simulink model "CT_tests_2020b"  (R2020b)
settings: Solver=ode4  StartTime=0.0  StopTime=0.4  FixedStep=10e-6  RelTol=1e-3
libraries: CT_RTDS x1, spsControlledCurrentSourceLib x1, spsSeriesRLCBranchLib x1, spspowerguiLib x1
settings Model: SimulationMode=accelerator  Creator=valeriytashchilin  LastModifiedBy=valeriytashchilin
settings DataIOCC: SaveOutput=off  SignalLogging=off  DSMLogging=off  SaveTime=off  ReturnWorkspaceOutputs=off

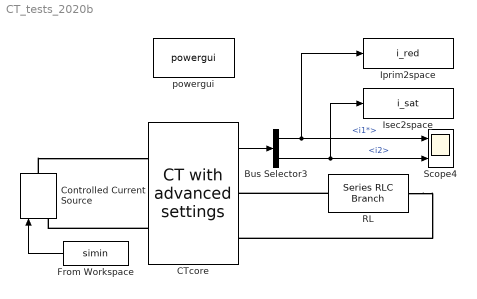
== system CT_tests_2020b ==
  Bus Selector3 : BusSelector  OutputSignals=i1*,i2
  CTcore : CT_RTDS/CT with advanced settings  Tag=CT  N1=2  N2=239  R2=0.48  L2=0  D=100  S=19.1e-4  Length=90e-2  Rloss=1e12  B0=0  c=0.08  k=4e-5  BETA1=0.96  ALFA=3e-5  Ms=1.7e6  a1=2550  a2=3150  a3=15000  b=2  SIMPLE=on  H2=600  DSCR=on  ts=-1  BAL=off
      settings: SourceProductName=CT RTDS
  Controlled Current Source : spsControlledCurrentSourceLib/Controlled Current Source  Initialize=on  Source_Type=AC  Amplitude=0  Phase=0  Frequency=0  Measurements=None
  From Workspace : FromWorkspace  VariableName=simin
  Iprim2space : ToWorkspace  VariableName=i_red  SaveFormat=Timeseries  SampleTime=-1
  Isec2space : ToWorkspace  VariableName=i_sat  SaveFormat=Timeseries  SampleTime=-1
  RL : spsSeriesRLCBranchLib/Series RLC Branch  LConnTagsString=__new0  RConnTagsString=__new0  BranchType=RL  Resistance=30/25  Inductance=30/25*0.6/(100*pi)  SetiL0=off  InitialCurrent=0  Capacitance=1e-6  Setx0=off  InitialVoltage=0  Measurements=None
  Scope4 : Scope  NumInputPorts=2
  powergui : spspowerguiLib/powergui  Priority=1  SimulationMode=Discrete  SampleTime=10e-6  frequency=60  Iterations=50  frequencyindice=0  Pbase=100e6  ErrMax=1e-4  UnitsV=kV  UnitsW=MW  buscounter=0  FunctionMessages=off  echomessages=off  EnableUseOfTLC=off  CurrentSourceSwitches=off  DisableSnubberDevices=off  DisableRonSwitches=off  DisableVfSwitches=off  DisplayEquations=off  AutomaticDiscreteSolvers=off  SolverType=Tustin/Backward Euler (TBE)  Interpol=off  ExternalGateDelay=off  methode=off  Ts=100  x0status=blocks  SPID=on  SwTol=0  HookPort=off  NonlinearTolerance=1e-4  nMaxIteration=100  ContinueOnMaxIteration=off  RestoreLinks=warning  ResistiveCurrentMeasurement=off  Frange=[0:2:500]  Ylog=off  Xlog=on  ShowGrid=off  save=off  variable=ZData  structure=0  ZoomFFT=off  StartTime=0.0  cycles=1  DisplayStyle=1  fundamental=60  FreqAxis=off  MaxFrequency=1000  frequencyindicesteady=1  RmsSteady=1  display=off
  wires:
  From Workspace/1 -> Controlled Current Source/1
  Bus Selector3/2 -> Isec2space/1, Scope4/2  "<i2>"
  Bus Selector3/1 -> Iprim2space/1, Scope4/1  "<i1*>"
  CTcore/1 -> Bus Selector3/1
  connections:
  RL/LConn1 -- CTcore/RConn1
  Controlled Current Source/RConn1 -- CTcore/LConn1
  CTcore/LConn2 -- Controlled Current Source/LConn1
  RL/RConn1 -- CTcore/RConn2
